simulink model "untitled"  (R2014a)
settings: Solver=ode45  StartTime=0.0  StopTime=8  RelTol=1e-3
settings Model: Creator=sh3787  LastModifiedBy=sh3787

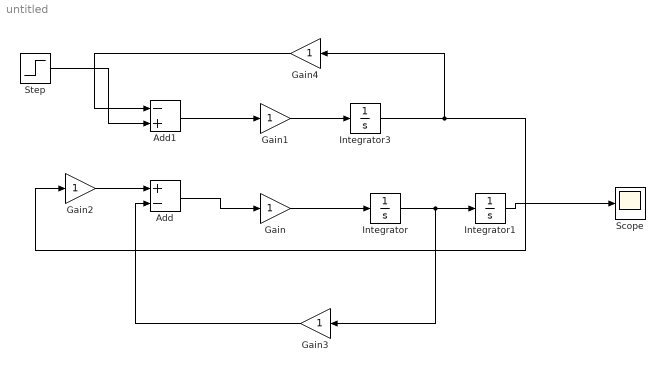
== system untitled ==
  Add : Sum  Inputs=+-
  Add1 : Sum  Inputs=-+
  Gain{,1..4} (5 alike) : Gain
  Integrator : Integrator
  Integrator1 : Integrator
  Integrator3 : Integrator
  Scope : Scope
      settings: TimeRange=1.069729286300246  YMin=6.831227436823106  YMax=6.944945848375452
  Step : Step  After=2  SampleTime=0
  wires:
  Gain/1 -> Integrator/1
  Gain1/1 -> Integrator3/1
  Integrator/1 -> Gain3/1, Integrator1/1
  Add/1 -> Gain/1
  Add1/1 -> Gain1/1
  Integrator3/1 -> Gain4/1, Gain2/1
  Gain2/1 -> Add/1
  Gain3/1 -> Add/2
  Step/1 -> Add1/2
  Gain4/1 -> Add1/1
  Integrator1/1 -> Scope/1
